simulink model "OxygenModel"  (R2024b)
settings: Solver=VariableStepAuto  StartTime=0.0  StopTime=100.0  RelTol=1e-3
libraries: simulink x1
settings Model: Creator=luima  LastModifiedBy=luima

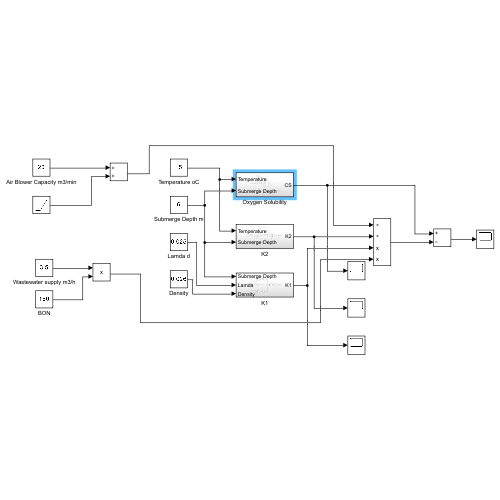
[thumbnail: Simulink's stored preview of the top-level diagram]
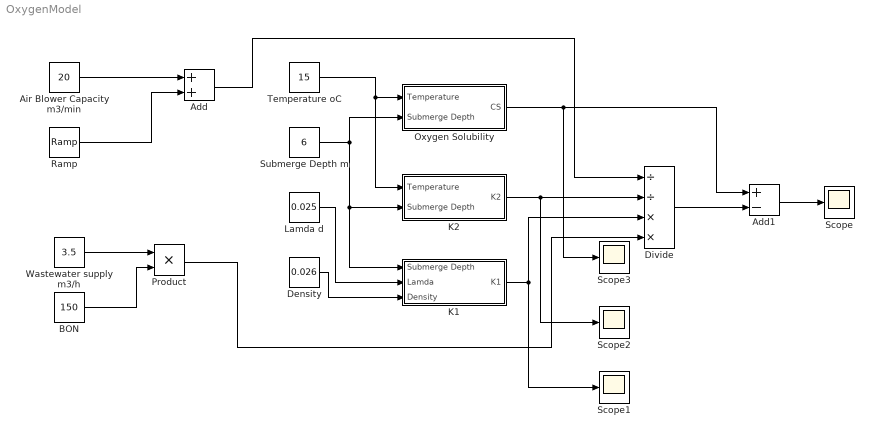
== system OxygenModel ==
  Add : Sum
  Add1 : Sum  Inputs=+-
  Air Blower Capacity m3/min : Constant  Value=20
  BON : Constant  Value=150
  Density : Constant  Value=0.026
  Divide : Product  Inputs=//**
  K1 : Subsystem
  K2 : Subsystem
  Lamda d : Constant  Value=0.025
  Oxygen Solubility : Subsystem
  Product : Product
  Ramp : simulink/Sources/Ramp  slope=2  start=0  InitialOutput=0
  Scope{,1..3} (4 alike) : Scope
  Submerge Depth m : Constant  Value=6
  Temperature oC : Constant  Value=15
  Wastewater supply m3/h : Constant  Value=3.5
  wires:
  Air Blower Capacity m3/min/1 -> Add/1
  Ramp/1 -> Add/2
  Temperature oC/1 -> Oxygen Solubility/1(Temperature), K2/1(Temperature)
  Submerge Depth m/1 -> K1/1(Submerge Depth), K2/2(Submerge Depth), Oxygen Solubility/2(Submerge Depth)
  Lamda d/1 -> K1/2(Lamda)
  Density/1 -> K1/3(Density)
  Wastewater supply m3/h/1 -> Product/1
  BON/1 -> Product/2
  Product/1 -> Divide/4
  K1/1(K1) -> Scope1/1, Divide/3
  K2/1(K2) -> Scope2/1, Divide/2
  Add/1 -> Divide/1
  Oxygen Solubility/1(CS) -> Scope3/1, Add1/1
  Divide/1 -> Add1/2
  Add1/1 -> Scope/1

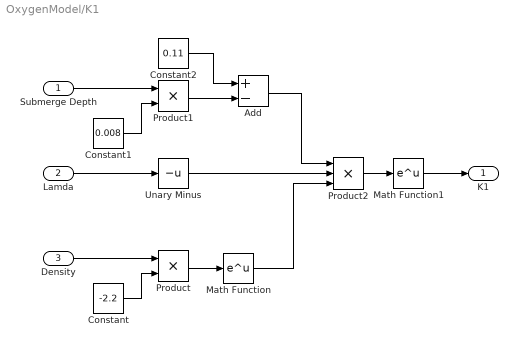
== system OxygenModel/K1 ==
  Submerge Depth : Inport
  Lamda : Inport  Port=2
  Density : Inport  Port=3
  Add : Sum  Inputs=+-
  Constant : Constant  Value=-2.2
  Constant1 : Constant  Value=0.008
  Constant2 : Constant  Value=0.11
  Math Function : Math
  Math Function1 : Math
  Product : Product
  Product1 : Product
  Product2 : Product  Inputs=3
  Unary Minus : UnaryMinus
  K1 : Outport
  wires:
  Constant/1 -> Product/2
  Density/1 -> Product/1
  Product/1 -> Math Function/1
  Constant1/1 -> Product1/2
  Submerge Depth/1 -> Product1/1
  Constant2/1 -> Add/1
  Product1/1 -> Add/2
  Lamda/1 -> Unary Minus/1
  Unary Minus/1 -> Product2/2
  Add/1 -> Product2/1
  Math Function/1 -> Product2/3
  Product2/1 -> Math Function1/1
  Math Function1/1 -> K1/1

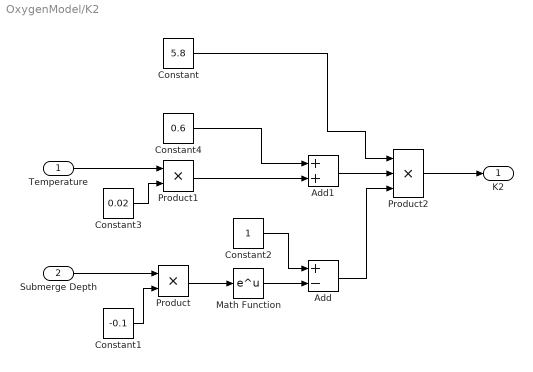
== system OxygenModel/K2 ==
  Temperature : Inport
  Submerge Depth : Inport  Port=2
  Add : Sum  Inputs=+-
  Add1 : Sum
  Constant : Constant  Value=5.8
  Constant1 : Constant  Value=-0.1
  Constant2 : Constant
  Constant3 : Constant  Value=0.02
  Constant4 : Constant  Value=0.6
  Math Function : Math
  Product : Product
  Product1 : Product
  Product2 : Product  Inputs=3
  K2 : Outport
  wires:
  Submerge Depth/1 -> Product/1
  Constant1/1 -> Product/2
  Product/1 -> Math Function/1
  Math Function/1 -> Add/2
  Constant2/1 -> Add/1
  Temperature/1 -> Product1/1
  Constant3/1 -> Product1/2
  Product1/1 -> Add1/2
  Constant4/1 -> Add1/1
  Constant/1 -> Product2/1
  Add1/1 -> Product2/2
  Add/1 -> Product2/3
  Product2/1 -> K2/1

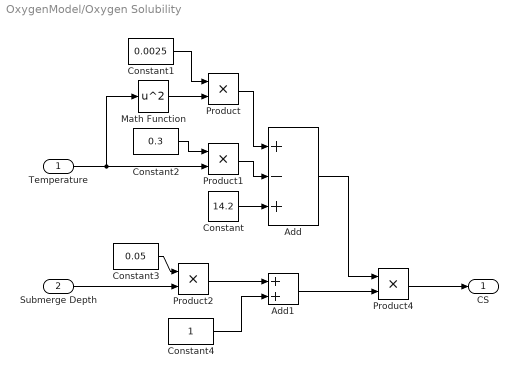
== system OxygenModel/Oxygen Solubility ==
  Temperature : Inport
  Submerge Depth : Inport  Port=2
  Add : Sum  Inputs=+-+
  Add1 : Sum
  Constant : Constant  Value=14.2
  Constant1 : Constant  Value=0.0025
  Constant2 : Constant  Value=0.3
  Constant3 : Constant  Value=0.05
  Constant4 : Constant
  Math Function : Math  Operator=square
  Product{,1..2,4} (4 alike) : Product
  CS : Outport
  wires:
  Constant/1 -> Add/3
  Temperature/1 -> Product1/2, Math Function/1
  Math Function/1 -> Product/2
  Constant1/1 -> Product/1
  Constant2/1 -> Product1/1
  Product1/1 -> Add/2
  Product/1 -> Add/1
  Constant3/1 -> Product2/1
  Submerge Depth/1 -> Product2/2
  Product2/1 -> Add1/1
  Constant4/1 -> Add1/2
  Add1/1 -> Product4/2
  Add/1 -> Product4/1
  Product4/1 -> CS/1
